simulink model "Simple_CDMA"  (Simulink 9.0)
settings: Solver=ode45  StartTime=0.0  StopTime=10.0  RelTol=1e-3  EnableMultiTasking=on
undefined symbols (not defined in the file): dfilt
libraries: commrandsrc2 x3, dspobslib x3, commsink2 x3, commnoisgen2 x1, commseqgen2 x1
settings Model: SuppressorTable=22 serialization::archive 11 0 6 0 0 0 0 0  Creator=changgang  LastModifiedBy=changgang
settings DataIOCC: LimitDataPoints=on  SignalLoggingSaveFormat=ModelDataLogs
settings OptimizationCC: InitFltsAndDblsToZero=on
settings DebuggingCC: SaveWithParameterizedLinksMsg=none  SignalResolutionControl=TryResolveAllWithWarning  SolverPrmCheckMsg=warning  MultiTaskDSMMsg=warning  MultiTaskCondExecSysMsg=none
settings GRTTargetCC: TargetFcnLib=ansi_tfl_tmw.mat  CombineOutputUpdateFcns=off  GRTInterface=on

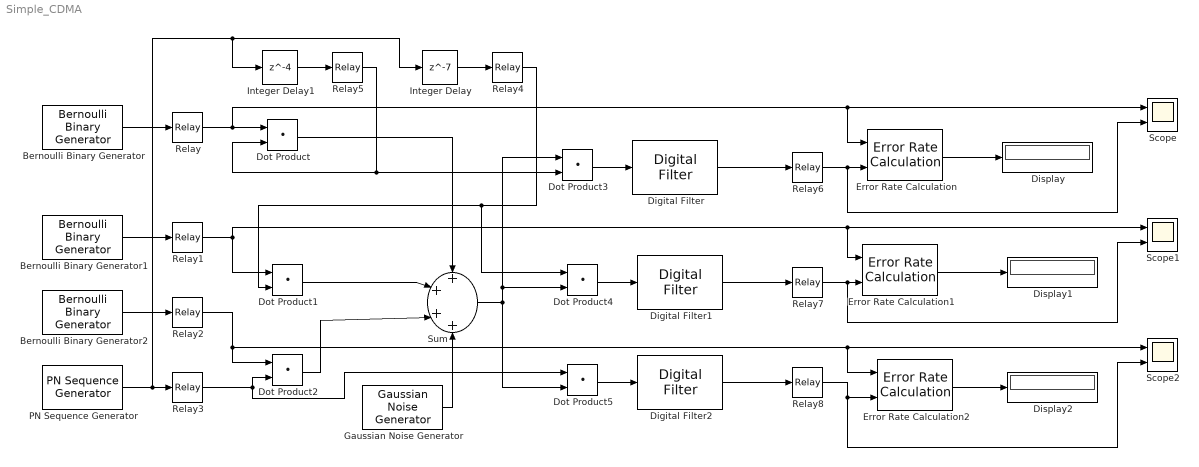
== system Simple_CDMA ==
  Bernoulli Binary Generator : commrandsrc2/Bernoulli Binary Generator  P=0.5  seed=61  Ts=0.5  frameBased=off  sampPerFrame=1  orient=off  outDataType=double
  Bernoulli Binary Generator1 : commrandsrc2/Bernoulli Binary Generator  P=0.5  seed=55  Ts=0.5  frameBased=off  sampPerFrame=1  orient=off  outDataType=double
  Bernoulli Binary Generator2 : commrandsrc2/Bernoulli Binary Generator  P=0.5  seed=36  Ts=0.5  frameBased=off  sampPerFrame=1  orient=off  outDataType=double
  Digital Filter : dspobslib/Digital Filter  TypePopup=IIR (poles & zeros)  IIRFiltStruct=Direct form II transposed  AllPoleFiltStruct=Direct form  FIRFiltStruct=Direct form  CoeffSource=Specify via dialog  NumCoeffs=[0.0004 0.0017 0.0025 0.0017 0.0004]  DenCoeffs=[1.0000 -3.1811 3.8623 -2.1130 0.4385]  BiQuadCoeffs=[1 0.3 0.4 1 0.1 0.2]  LatticeCoeffs=[0.2 0.4]  denIgnore=on  FiltPerSampPopup=One filter per frame  IC=0  ICnum=0  ICden=0  roundingMode=Floor  overflowMode=off  ScaleValues=1  scaleValueFracLength=14  stageInFracLength=15  stageOutFracLength=15  FilterSource=Specify via dialog  dfiltObjectName=dfilt.dffir([1 2 1])  InputProcessing=Inherited (this choice will be removed - see release notes)
      settings: SourceProductName=DSP System Toolbox  SourceProductBaseCode=DS
  Digital Filter1 : dspobslib/Digital Filter  TypePopup=IIR (poles & zeros)  IIRFiltStruct=Direct form II transposed  AllPoleFiltStruct=Direct form  FIRFiltStruct=Direct form  CoeffSource=Specify via dialog  NumCoeffs=[0.0004 0.0017 0.0025 0.0017 0.0004]  DenCoeffs=[1.0000 -3.1811 3.8623 -2.1130 0.4385]  BiQuadCoeffs=[1 0.3 0.4 1 0.1 0.2]  LatticeCoeffs=[0.2 0.4]  denIgnore=on  FiltPerSampPopup=One filter per frame  IC=0  ICnum=0  ICden=0  roundingMode=Floor  overflowMode=off  ScaleValues=1  scaleValueFracLength=14  stageInFracLength=15  stageOutFracLength=15  FilterSource=Specify via dialog  dfiltObjectName=dfilt.dffir([1 2 1])  InputProcessing=Inherited (this choice will be removed - see release notes)
      settings: SourceProductName=DSP System Toolbox  SourceProductBaseCode=DS
  Digital Filter2 : dspobslib/Digital Filter  TypePopup=IIR (poles & zeros)  IIRFiltStruct=Direct form II transposed  AllPoleFiltStruct=Direct form  FIRFiltStruct=Direct form  CoeffSource=Specify via dialog  NumCoeffs=[0.0004 0.0017 0.0025 0.0017 0.0004]  DenCoeffs=[1.0000 -3.1811 3.8623 -2.1130 0.4385]  BiQuadCoeffs=[1 0.3 0.4 1 0.1 0.2]  LatticeCoeffs=[0.2 0.4]  denIgnore=on  FiltPerSampPopup=One filter per frame  IC=0  ICnum=0  ICden=0  roundingMode=Floor  overflowMode=off  ScaleValues=1  scaleValueFracLength=14  stageInFracLength=15  stageOutFracLength=15  FilterSource=Specify via dialog  dfiltObjectName=dfilt.dffir([1 2 1])  InputProcessing=Inherited (this choice will be removed - see release notes)
      settings: SourceProductName=DSP System Toolbox  SourceProductBaseCode=DS
  Display : Display
  Display1 : Display
  Display2 : Display
  Dot Product{,1..5} (6 alike) : DotProduct  InputSameDT=on  OutDataTypeStr=Inherit: Inherit via internal rule
  Error Rate Calculation : commsink2/Error Rate Calculation  N=0  st_delay=0  cp_mode=Entire frame  subframe=[]  PMode=Port  WsName=ErrorVec  RsMode2=off  stop=off  numErr=100  maxBits=1e6
  Error Rate Calculation1 : commsink2/Error Rate Calculation  N=0  st_delay=0  cp_mode=Entire frame  subframe=[]  PMode=Port  WsName=ErrorVec  RsMode2=off  stop=off  numErr=100  maxBits=1e6
  Error Rate Calculation2 : commsink2/Error Rate Calculation  N=0  st_delay=0  cp_mode=Entire frame  subframe=[]  PMode=Port  WsName=ErrorVec  RsMode2=off  stop=off  numErr=100  maxBits=1e6
  Gaussian Noise Generator : commnoisgen2/Gaussian Noise Generator  m=0  d=0.001  s=61  Ts=0.01  frameBased=off  sampPerFrame=1  orient=off  outDataType=double
  Integer Delay : Delay  DelayLength=7  InputProcessing=Inherited
  Integer Delay1 : Delay  DelayLength=4  InputProcessing=Inherited
  PN Sequence Generator : commseqgen2/PN Sequence Generator  poly=[1 1 0 0 1]  ini_sta=[0 1 0 0]  outBitMaskSource=Dialog parameter  shift=0  outVarSiz=off  maxOutSizeMode=Dialog parameter  maxOutSize=[10 1]  Ts=0.01  frameBased=off  sampPerFrame=1  reset=off  bitPackedOutputs=off  outDataType=double  numPackedBits=8  bitPackDataSigned=off  bitPackedOutDType=double
  Relay : Relay  OnSwitchValue=0.9  OffSwitchValue=0.1  OffOutputValue=-1  SampleTime=0.5
  Relay1 : Relay  OnSwitchValue=0.9  OffSwitchValue=0.1  OffOutputValue=-1  SampleTime=0.5
  Relay2 : Relay  OnSwitchValue=0.9  OffSwitchValue=0.1  OffOutputValue=-1  SampleTime=0.5
  Relay3 : Relay  OffOutputValue=-1  SampleTime=0.01
  Relay4 : Relay  OffOutputValue=-1  SampleTime=0.01
  Relay5 : Relay  OffOutputValue=-1  SampleTime=0.01
  Relay6 : Relay  OnSwitchValue=0.51  OffSwitchValue=0.49  OffOutputValue=-1  SampleTime=0.5
  Relay7 : Relay  OnSwitchValue=0.51  OffSwitchValue=0.49  OffOutputValue=-1  SampleTime=0.5
  Relay8 : Relay  OnSwitchValue=0.51  OffSwitchValue=0.49  OffOutputValue=-1  SampleTime=0.5
  Scope : Scope  NumInputPorts=2
  Scope1 : Scope  NumInputPorts=2
  Scope2 : Scope  NumInputPorts=2
  Sum : Sum  Inputs=+||+||+||+
  wires:
  Bernoulli Binary Generator/1 -> Relay/1
  Relay/1 -> Dot Product/1, Scope/1, Error Rate Calculation/1
  Dot Product/1 -> Sum/1
  Bernoulli Binary Generator1/1 -> Relay1/1
  Relay1/1 -> Dot Product1/1, Scope1/1, Error Rate Calculation1/1
  Bernoulli Binary Generator2/1 -> Relay2/1
  Relay2/1 -> Dot Product2/1, Scope2/1, Error Rate Calculation2/1
  PN Sequence Generator/1 -> Integer Delay1/1, Integer Delay/1, Relay3/1
  Integer Delay/1 -> Relay4/1
  Integer Delay1/1 -> Relay5/1
  Relay3/1 -> Dot Product5/1, Dot Product2/2
  Relay4/1 -> Dot Product1/2, Dot Product4/1
  Relay5/1 -> Dot Product/2, Dot Product3/2
  Relay6/1 -> Error Rate Calculation/2, Scope/2
  Error Rate Calculation/1 -> Display/1
  Error Rate Calculation1/1 -> Display1/1
  Error Rate Calculation2/1 -> Display2/1
  Relay7/1 -> Error Rate Calculation1/2, Scope1/2
  Relay8/1 -> Scope2/2, Error Rate Calculation2/2
  Dot Product2/1 -> Sum/3
  Dot Product1/1 -> Sum/2
  Gaussian Noise Generator/1 -> Sum/4
  Sum/1 -> Dot Product3/1, Dot Product4/2, Dot Product5/2
  Dot Product3/1 -> Digital Filter/1
  Dot Product4/1 -> Digital Filter1/1
  Dot Product5/1 -> Digital Filter2/1
  Digital Filter/1 -> Relay6/1
  Digital Filter1/1 -> Relay7/1
  Digital Filter2/1 -> Relay8/1
